simulink model "SWT_fullModel_final"  (R2023b)
settings: Solver=FixedStepAuto  StartTime=0.0  StopTime=329  RelTol=1e-3
values from neighbouring files (symbols this model uses):
  A = 19.76    [init_SWT_final.m]
  alpha = 0.19    [init_SWT_final.m]
  Cf = 1e-6    (= 1e-06)    [init_SWT_final.m]
  Cg_half = 36e-6    (= 3.6e-05)    [init_SWT_final.m]
  Cp_half = 0.8e-6    (= 8e-07)    [init_SWT_final.m]
  D_eq = 1500    [init_SWT_final.m]
  gearbox_ratio = 8.27    [init_SWT_final.m]
  J_g = 0.0491    [init_SWT_final.m]
  J_r = 142.99    [init_SWT_final.m]
  K_eq = 16887    [init_SWT_final.m]
  Lg = 12e-3    (= 0.012)    [init_SWT_final.m]
  LsLm = 3.75e-3    (= 0.00375)    [init_SWT_final.m]
  n_pp = 2    [init_SWT_final.m]
  r_rot = sqrt(A/pi)    [init_SWT_final.m]
  Rg = 2    [init_SWT_final.m]
  rho = 1.225    [init_SWT_final.m]
  Rlp1 = 100    [init_SWT_final.m]
  Rlp2 = 74    [init_SWT_final.m]
  RsRm = 2.49    [init_SWT_final.m]
  T_rated = n_eff_gen*5800/w_r_rated    [init_SWT_final.m]
  Ug = 400    [init_SWT_final.m]
  z = 12    [init_SWT_final.m]
  z_ref = 12    [init_SWT_final.m]
libraries: spsThreePhaseSeriesRLCBranchLib x9, spsRMSLib x6, spsThreePhaseVIMeasurementLib x4, spsGroundLib x3, dspstat3 x3, spsPower3phInstantaneousLib x3, spsSeriesRLCBranchLib x2, spsThreePhaseParallelRLCLoadLib x2, simulink x2, spsAsynchronousMachineSIUnitsLib x1, spsThreePhaseSourceLib x1, spspowerguiLib x1
settings Model: Creator=leons  LastModifiedBy=leons
settings DataIOCC: LoggingToFile=on

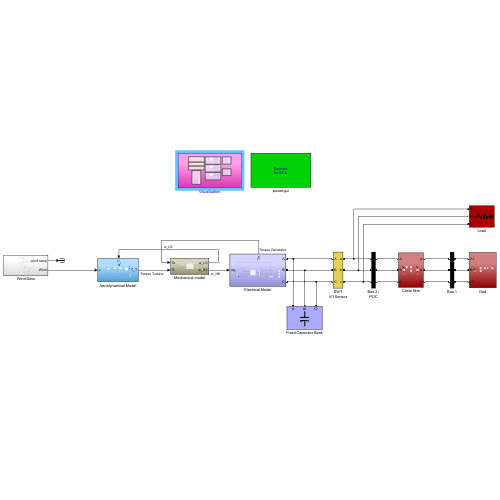
[thumbnail: Simulink's stored preview of the top-level diagram]
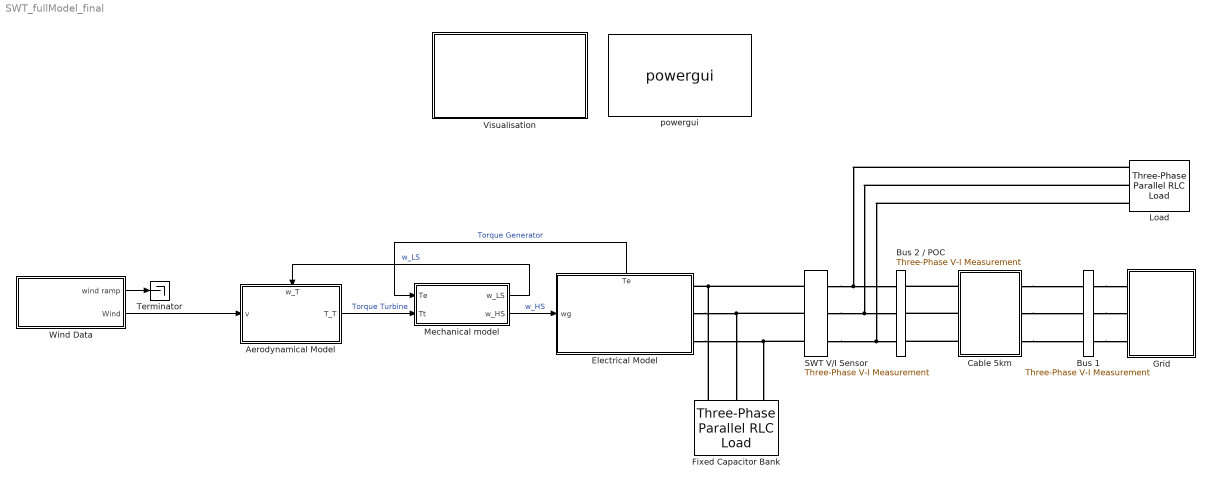
== system SWT_fullModel_final ==
  Aerodynamical Model : Subsystem
      settings: PortSchema="{\"entries\":[{\"content\":{\"sides\":[{\"content\":{\"connectorIds\":[\"In1\"]},\"type\":\"ConnectorPlacement.EquallySpacedRectSide\",\"uuid\":\"ecf32035-92b1-4f8a-b97d-d3e4d481fbcb\"},{\"content\":{\"connectorIds\":[\"Out1\"],\"side\":\"RIGHT\"},\"type\":\"ConnectorPlacement.EquallySpacedRectSide\",\"uuid\":\"1e721a83-f5e0-4c63-8c71-e92131e65c4e\"},{\"content\":{\"connectorIds\":[\"In2\"],\"side\":\"TOP\"},\"type\":\"ConnectorPlacement.EquallySpacedRectSide\",\"uuid\":\"951b011d-70ba-4a70-99b1-ab34aaa137eb\"}]},\"type\":\"ConnectorPlacement.EquallySpacedConnector\",\"uuid\":\"fe5cab3d-0189-4813-bb49-ec0d1ef7e469\"}],\"packageUris\":[\"http://schema.mathworks.com/mf0/Connector/R2020b\"],\"version\":\"1.0\"}"
  Bus 1 : spsThreePhaseVIMeasurementLib/Three-Phase V-I Measurement  VoltageMeasurement=phase-to-ground  SetLabelV=on  LabelV=Vabc_bus1  Vpu=off  VpuLL=off  CurrentMeasurement=yes  SetLabelI=on  LabelI=Iabc_bus1  Ipu=off  Pbase=100e6  Vbase=500e3  OutputType=Complex  PhasorSimulation=off  PSBequivalent=0
  Bus 2 / POC : spsThreePhaseVIMeasurementLib/Three-Phase V-I Measurement  VoltageMeasurement=phase-to-ground  SetLabelV=on  LabelV=Vabc_bus2  Vpu=off  VpuLL=off  CurrentMeasurement=yes  SetLabelI=on  LabelI=Iabc_bus2  Ipu=off  Pbase=100e6  Vbase=500e3  OutputType=Complex  PhasorSimulation=off  PSBequivalent=0
  Cable 5km : Subsystem
  Electrical Model : Subsystem
      settings: PortSchema="{\"entries\":[{\"content\":{\"sides\":[{\"content\":{\"connectorIds\":[\"In1\"]},\"type\":\"ConnectorPlacement.EquallySpacedRectSide\",\"uuid\":\"9f37345d-f4a4-45e1-920f-d9c37b4ca0b7\"},{\"content\":{\"connectorIds\":[\"RConn1\",\"RConn2\",\"RConn3\"],\"side\":\"RIGHT\"},\"type\":\"ConnectorPlacement.EquallySpacedRectSide\",\"uuid\":\"4b2a57c5-bb37-44b9-8bd5-b50d4c851d22\"},{\"content\":{\"connectorIds\":[\"Out1\"],\"side\":\"TOP\"},\"type\":\"ConnectorPlacement.EquallySpacedRectSide\",\"uuid\":\"91cf862d-bae5-40ba-b973-5330e4f84dcc\"}]},\"type\":\"ConnectorPlacement.EquallySpacedConnector\",\"uuid\":\"d5ba1b97-1505-48bd-9b20-6cd61836b2e9\"}],\"packageUris\":[\"http://schema.mathworks.com/mf0/Connector/R2020b\"],\"version\":\"1.0\"}"
  Fixed Capacitor Bank : spsThreePhaseParallelRLCLoadLib/Three-Phase Parallel RLC Load  LConnTagsString=A|B|C  Configuration=Delta  NominalVoltage=V_nominal  Vabc=[1e3 1e3 1e3]  Vabcp=[1e3 1e3 1e3]  NominalFrequency=fs  UnbalancedPower=off  ActivePower=0  InductivePower=0  CapacitivePower=Q_comp_real  Pabc=[10e3 9e3 11e3]  QLabc=[100 90 110]  QCabc=[100 90 110]  Pabcp=[10e3 9e3 11e3]  QLabcp=[100 90 110]  QCabcp=[100 90 110]  Measurements=None  LoadType=constant Z
  Grid : Subsystem
  Load : spsThreePhaseParallelRLCLoadLib/Three-Phase Parallel RLC Load  LConnTagsString=A|B|C  Configuration=Y (grounded)  NominalVoltage=400  Vabc=[1e3 1e3 1e3]  Vabcp=[1e3 1e3 1e3]  NominalFrequency=50  UnbalancedPower=off  ActivePower=Load_at_POC  InductivePower=0  CapacitivePower=0  Pabc=[10e3 9e3 11e3]  QLabc=[100 90 110]  QCabc=[100 90 110]  Pabcp=[10e3 9e3 11e3]  QLabcp=[100 90 110]  QCabcp=[100 90 110]  Measurements=None  LoadType=constant Z
  Mechanical model : Subsystem
  SWT V/I Sensor : spsThreePhaseVIMeasurementLib/Three-Phase V-I Measurement  VoltageMeasurement=phase-to-ground  SetLabelV=on  LabelV=Vabc_SWT  Vpu=off  VpuLL=off  CurrentMeasurement=yes  SetLabelI=on  LabelI=Iabc_SWT  Ipu=off  Pbase=100e6  Vbase=500e3  OutputType=Complex  PhasorSimulation=off  PSBequivalent=0
  Terminator : Terminator
  Visualisation : Subsystem
  Wind Data : Subsystem
  powergui : spspowerguiLib/powergui  Priority=1  SimulationMode=Discrete  SampleTime=50e-6  frequency=60  Iterations=50  frequencyindice=50  Pbase=100e6  ErrMax=1e-4  UnitsV=kV  UnitsW=MW  buscounter=2  FunctionMessages=off  echomessages=off  EnableUseOfTLC=off  CurrentSourceSwitches=off  DisableSnubberDevices=off  DisableRonSwitches=off  DisableVfSwitches=off  DisplayEquations=off  AutomaticDiscreteSolvers=off  SolverType=Tustin/Backward Euler (TBE)  Interpol=off  ExternalGateDelay=off  methode=off  Ts=100  x0status=blocks  SPID=on  SwTol=0  HookPort=off  NonlinearTolerance=1e-4  nMaxIteration=100  ContinueOnMaxIteration=off  RestoreLinks=warning  ResistiveCurrentMeasurement=off  Frange=[0:2:500]  Ylog=off  Xlog=on  ShowGrid=off  save=off  variable=ZData  structure=0  ZoomFFT=off  StartTime=0.0  cycles=1  DisplayStyle=1  fundamental=60  FreqAxis=off  MaxFrequency=1000  frequencyindicesteady=1  RmsSteady=1  display=off
  wires:
  Mechanical model/1(w_LS) -> Aerodynamical Model/2(w_T)  "w_LS"
  Aerodynamical Model/1(T_T) -> Mechanical model/2(Tt)  "Torque Turbine"
  Mechanical model/2(w_HS) -> Electrical Model/1(wg)  "w_HS"
  Electrical Model/1("Te ") -> Mechanical model/1(Te)  "Torque Generator"
  Wind Data/2(Wind) -> Aerodynamical Model/1(v)
  Wind Data/1(wind ramp) -> Terminator/1
  connections:
  Electrical Model/RConn3 -- Fixed Capacitor Bank/LConn3 -- SWT V/I Sensor/LConn3
  Load/LConn2 -- Bus 2 / POC/LConn2 -- SWT V/I Sensor/RConn2
  Load/LConn1 -- Bus 2 / POC/LConn1 -- SWT V/I Sensor/RConn1
  Bus 1/RConn1 -- Grid/LConn1
  Bus 1/RConn2 -- Grid/LConn2
  Bus 1/RConn3 -- Grid/LConn3
  Load/LConn3 -- SWT V/I Sensor/RConn3 -- Bus 2 / POC/LConn3
  Electrical Model/RConn2 -- Fixed Capacitor Bank/LConn2 -- SWT V/I Sensor/LConn2
  Fixed Capacitor Bank/LConn1 -- SWT V/I Sensor/LConn1 -- Electrical Model/RConn1
  Cable 5km/RConn1 -- Bus 1/LConn1
  Cable 5km/RConn2 -- Bus 1/LConn2
  Cable 5km/RConn3 -- Bus 1/LConn3
  Cable 5km/LConn1 -- Bus 2 / POC/RConn1
  Cable 5km/LConn2 -- Bus 2 / POC/RConn2
  Cable 5km/LConn3 -- Bus 2 / POC/RConn3

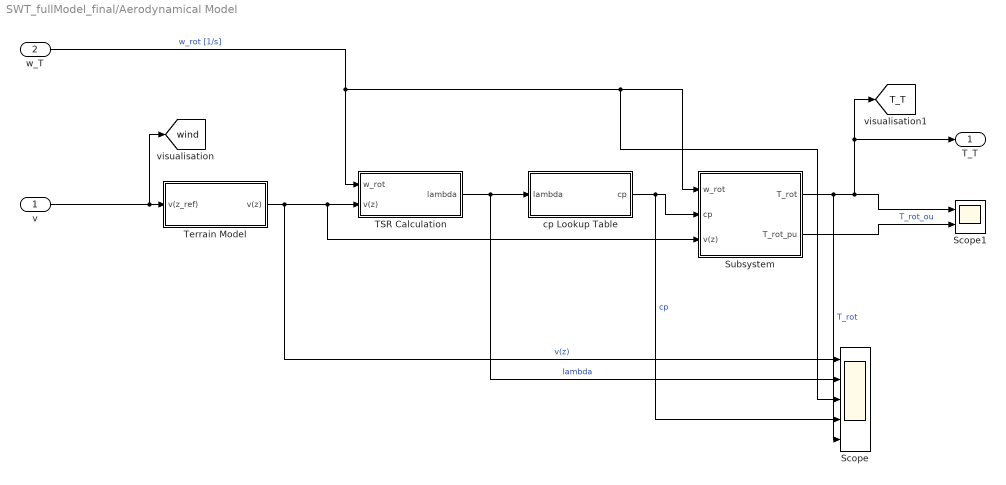
== system SWT_fullModel_final/Aerodynamical Model ==
  v : Inport
  w_T : Inport  Port=2
  Scope : Scope  NumInputPorts=5
  Scope1 : Scope  NumInputPorts=2
  Subsystem : Subsystem
  TSR Calculation : Subsystem
  Terrain Model : Subsystem
  cp Lookup Table : Subsystem
  T_T : Outport
  tag scope: T_T=global, wind=global
  wires:
  Terrain Model/1(v(z)) -> Scope/1, Subsystem/3(v(z)), TSR Calculation/2(v(z))  "v(z)"
  cp Lookup Table/1(cp) -> Scope/4, Subsystem/2(cp)  "cp"
  w_T/1 -> TSR Calculation/1(w_rot), Scope/3, Subsystem/1(w_rot)  "w_rot [1/s]"
  TSR Calculation/1(lambda) -> Scope/2, cp Lookup Table/1(lambda)  "lambda"
  Subsystem/2(T_rot_pu) -> Scope1/2  "T_rot_ou"
  v/1 -> [wind], Terrain Model/1(v(z_ref))
  Subsystem/1(T_rot) -> Scope/5, [T_T], T_T/1, Scope1/1  "T_rot"

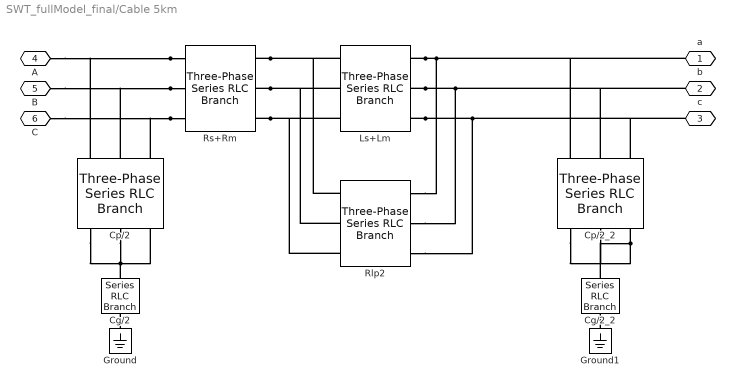
== system SWT_fullModel_final/Cable 5km ==
  Cg/2 : spsSeriesRLCBranchLib/Series RLC Branch  LConnTagsString=__new0  RConnTagsString=__new0  BranchType=C  Resistance=1  Inductance=1e-3  SetiL0=off  InitialCurrent=0  Capacitance=Cg_half  Setx0=off  InitialVoltage=0  Measurements=None
  Cg/2_2 : spsSeriesRLCBranchLib/Series RLC Branch  LConnTagsString=__new0  RConnTagsString=__new0  BranchType=C  Resistance=1  Inductance=1e-3  SetiL0=off  InitialCurrent=0  Capacitance=Cg_half  Setx0=off  InitialVoltage=0  Measurements=None
  Cp/2 : spsThreePhaseSeriesRLCBranchLib/Three-Phase Series RLC Branch  LConnTagsString=A|B|C  RConnTagsString=A|B|C  BranchType=C  Resistance=10  Inductance=12e-3  Capacitance=Cp_half  Measurements=None
  Cp/2_2 : spsThreePhaseSeriesRLCBranchLib/Three-Phase Series RLC Branch  LConnTagsString=A|B|C  RConnTagsString=A|B|C  BranchType=C  Resistance=10  Inductance=12e-3  Capacitance=Cp_half  Measurements=None
  Ground : spsGroundLib/Ground  LConnTagsString=a
  Ground1 : spsGroundLib/Ground  LConnTagsString=a
  Ls+Lm : spsThreePhaseSeriesRLCBranchLib/Three-Phase Series RLC Branch  LConnTagsString=A|B|C  RConnTagsString=A|B|C  BranchType=L  Resistance=1.28  Inductance=LsLm  Capacitance=1e-6  Measurements=None
  Rlp2 : spsThreePhaseSeriesRLCBranchLib/Three-Phase Series RLC Branch  LConnTagsString=A|B|C  RConnTagsString=A|B|C  BranchType=R  Resistance=Rlp2  Inductance=12e-3  Capacitance=1e-6  Measurements=None
  Rs+Rm : spsThreePhaseSeriesRLCBranchLib/Three-Phase Series RLC Branch  LConnTagsString=A|B|C  RConnTagsString=A|B|C  BranchType=R  Resistance=RsRm  Inductance=12e-3  Capacitance=1e-6  Measurements=None
  a : PMIOPort  Side=Right
  b : PMIOPort  Port=2  Side=Right
  c : PMIOPort  Port=3  Side=Right
  A : PMIOPort  Port=4  Side=Left
  B : PMIOPort  Port=5  Side=Left
  C : PMIOPort  Port=6  Side=Left
  connections:
  Ground1/LConn1 -- Cg/2_2/RConn1
  Cp/2_2/RConn3 -- Cg/2_2/LConn1 -- Cp/2_2/RConn2 -- Cp/2_2/RConn1
  Ground/LConn1 -- Cg/2/RConn1
  Cp/2/RConn2 -- Cg/2/LConn1 -- Cp/2/RConn3 -- Cp/2/RConn1
  Rs+Rm/LConn1 -- Cp/2/LConn1 -- A/RConn1
  Rs+Rm/LConn2 -- Cp/2/LConn2 -- B/RConn1
  Rs+Rm/LConn3 -- Cp/2/LConn3 -- C/RConn1
  Ls+Lm/RConn3 -- c/RConn1 -- Cp/2_2/LConn3 -- Rlp2/RConn3
  Ls+Lm/RConn2 -- b/RConn1 -- Cp/2_2/LConn2 -- Rlp2/RConn2
  Ls+Lm/RConn1 -- a/RConn1 -- Cp/2_2/LConn1 -- Rlp2/RConn1
  Rs+Rm/RConn3 -- Rlp2/LConn3 -- Ls+Lm/LConn3
  Rs+Rm/RConn2 -- Rlp2/LConn2 -- Ls+Lm/LConn2
  Rs+Rm/RConn1 -- Rlp2/LConn1 -- Ls+Lm/LConn1

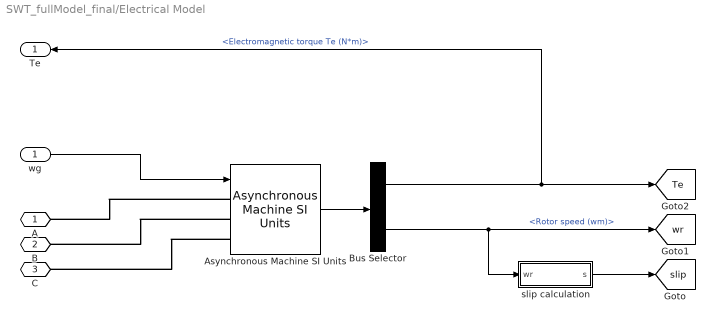
== system SWT_fullModel_final/Electrical Model ==
  wg : Inport
  Asynchronous Machine SI Units : spsAsynchronousMachineSIUnitsLib/Asynchronous Machine SI Units  RotorType=Squirrel-cage  PresetModel=No  MechanicalLoad=Speed w  ShowDetailedParameters=on  ReferenceFrame=Synchronous  Units=SI  MeasurementBus=off  NominalParameters=[5500 400 50]  VoltageRatio=1  Stator=[1.09445 0.00442]  Rotor=[1.0676 0.00442]  Cage1=[0.4155 0.002066]  Cage2=[0.4168 0.0003495]  Lm=0.14815  Mechanical=[0.0131 0.002985 2]  PolePairs=2  InitialConditions=[0 0 5.46772 5.46772 5.46772 -86.7675 -206.767 33.2325]  SimulateSaturation=off  Saturation=[14.03593122, 27.81365428, 53.79336849, 72.68890987, 97.98006896, 148.6815601, 215.7428561, 302.9841135, 428.7778367 ; 230, 322, 414, 460, 506, 552, 598, 644, 690]  LoadFlowParameters=0  TsPowergui=0  TsBlock=-1  IterativeModel=Trapezoidal non iterative  IterativeDiscreteModel=Trapezoidal non iterative  Pmec=0
  Bus Selector : BusSelector  OutputSignals=Mechanical.Electromagnetic torque Te (N*m),Mechanical.Rotor speed (wm)
  slip calculation : Subsystem
  A : PMIOPort  Side=Right
  B : PMIOPort  Port=2  Side=Right
  C : PMIOPort  Port=3  Side=Right
  "Te " : Outport
  tag scope: Te=global, slip=global, wr=global
  wires:
  Asynchronous Machine SI Units/1 -> Bus Selector/1
  wg/1 -> Asynchronous Machine SI Units/1
  Bus Selector/1 -> "Te "/1, [Te]  "<Electromagnetic torque Te (N*m)>"
  Bus Selector/2 -> slip calculation/1(wr), [wr]  "<Rotor speed (wm)>"
  slip calculation/1(s) -> [slip]
  connections:
  Asynchronous Machine SI Units/LConn2 -- B/RConn1
  Asynchronous Machine SI Units/LConn1 -- A/RConn1
  Asynchronous Machine SI Units/LConn3 -- C/RConn1

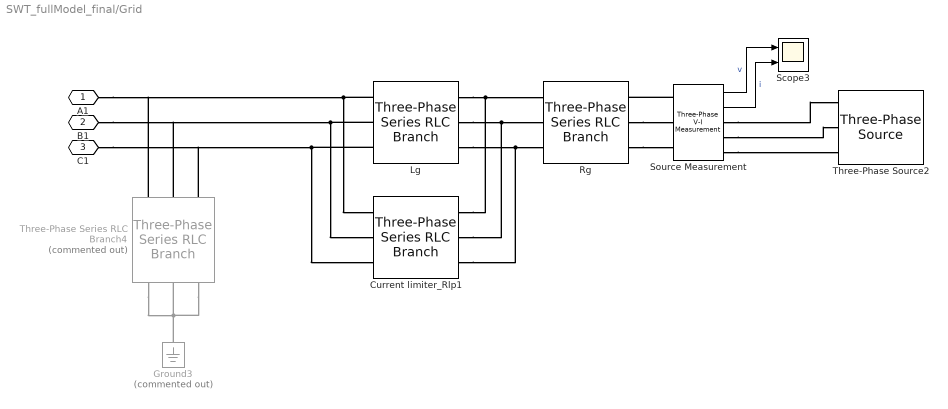
== system SWT_fullModel_final/Grid ==
  Current limiter_Rlp1 : spsThreePhaseSeriesRLCBranchLib/Three-Phase Series RLC Branch  LConnTagsString=A|B|C  RConnTagsString=A|B|C  BranchType=R  Resistance=Rlp1  Inductance=1e-3  Capacitance=1e-6  Measurements=None
  Ground3 : spsGroundLib/Ground  Commented=on  LConnTagsString=a
  Lg : spsThreePhaseSeriesRLCBranchLib/Three-Phase Series RLC Branch  LConnTagsString=A|B|C  RConnTagsString=A|B|C  BranchType=L  Resistance=200  Inductance=Lg  Capacitance=1e-6  Measurements=None
  Rg : spsThreePhaseSeriesRLCBranchLib/Three-Phase Series RLC Branch  LConnTagsString=A|B|C  RConnTagsString=A|B|C  BranchType=R  Resistance=Rg  Inductance=1e-3  Capacitance=1e-6  Measurements=None
  Scope3 : Scope  NumInputPorts=2
  Source Measurement : spsThreePhaseVIMeasurementLib/Three-Phase V-I Measurement  VoltageMeasurement=phase-to-phase  SetLabelV=off  LabelV=Vabc  Vpu=off  VpuLL=off  CurrentMeasurement=yes  SetLabelI=off  LabelI=Iabc  Ipu=off  Pbase=100e6  Vbase=500e3  OutputType=Complex  PhasorSimulation=off  PSBequivalent=0
  Three-Phase Series RLC Branch4 : spsThreePhaseSeriesRLCBranchLib/Three-Phase Series RLC Branch  Commented=on  LConnTagsString=A|B|C  RConnTagsString=A|B|C  BranchType=C  Resistance=2  Inductance=1e-3  Capacitance=Cf  Measurements=None
  Three-Phase Source2 : spsThreePhaseSourceLib/Three-Phase Source  InternalConnection=Yg  VoltagePhases=off  Voltage=Ug  PhaseAngle=0  Voltage_phases=[25e3 25e3 25e3]/sqrt(3)  PhaseAngles_phases=[0 -120 +120]  Frequency=50  NonIdealSource=off  SpecifyImpedance=off  Resistance=5.17  Inductance=12e-3  ShortCircuitLevel=100e6  BaseVoltage=400  XRratio=0.73  BusType=swing  Pref=10e3  Qref=0  Prefabc=[10e3, 10e3, 10e3]  Qrefabc=[0, 0, 0]  Qmin=-inf  Qmax=inf
  A1 : PMIOPort  Side=Left
  B1 : PMIOPort  Port=2  Side=Left
  C1 : PMIOPort  Port=3  Side=Left
  wires:
  Source Measurement/2 -> Scope3/2  "i"
  Source Measurement/1 -> Scope3/1  "v"
  connections:
  Lg/RConn2 -- Current limiter_Rlp1/RConn2 -- Rg/LConn2
  Lg/LConn1 -- Three-Phase Series RLC Branch4/LConn1 -- A1/RConn1 -- Current limiter_Rlp1/LConn1
  Lg/RConn3 -- Current limiter_Rlp1/RConn3 -- Rg/LConn3
  Lg/RConn1 -- Current limiter_Rlp1/RConn1 -- Rg/LConn1
  Lg/LConn3 -- Three-Phase Series RLC Branch4/LConn3 -- C1/RConn1 -- Current limiter_Rlp1/LConn3
  Lg/LConn2 -- Three-Phase Series RLC Branch4/LConn2 -- B1/RConn1 -- Current limiter_Rlp1/LConn2
  Source Measurement/RConn3 -- Three-Phase Source2/RConn3
  Rg/RConn2 -- Source Measurement/LConn2
  Rg/RConn3 -- Source Measurement/LConn3
  Source Measurement/RConn2 -- Three-Phase Source2/RConn2
  Source Measurement/RConn1 -- Three-Phase Source2/RConn1
  Source Measurement/LConn1 -- Rg/RConn1
  Ground3/LConn1 -- Three-Phase Series RLC Branch4/RConn3 -- Three-Phase Series RLC Branch4/RConn2 -- Three-Phase Series RLC Branch4/RConn1

== system SWT_fullModel_final/Mechanical model ==
  Te : Inport
  Tt : Inport  Port=2
  2 Mass Model : Subsystem
  Gain1 : Gain  Gain=gearbox_ratio
  Gain2 : Gain  Gain=gearbox_ratio
  Gain3 : Gain  Gain=-1
  w_LS : Outport
  w_HS : Outport  Port=2
  tag scope: w_HS=global, w_LS=global
  wires:
  Tt/1 -> 2 Mass Model/2(T_turbine)  "T_turbine"
  Te/1 -> Gain3/1  "T_generator"
  2 Mass Model/1(w_T) -> [w_LS], w_LS/1  "w_LS"
  2 Mass Model/2(w_G) -> Gain2/1
  Gain1/1 -> 2 Mass Model/1(T_generator)
  Gain3/1 -> Gain1/1
  Gain2/1 -> w_HS/1, [w_HS]  "w_HS"

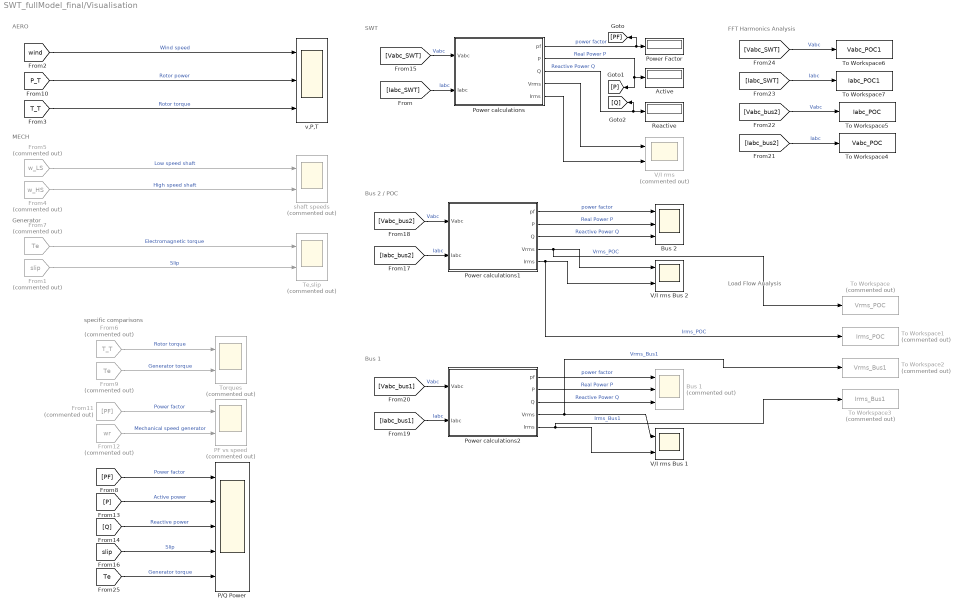
== system SWT_fullModel_final/Visualisation ==
  note: FFT Harmonics Analysis
  note: specific comparisons
  note: AERO
  note: MECH
  note: Generator
  note: SWT
  note: Bus 2 / POC
  note: Bus 1
  note: Load Flow Analysis
  Active : Display
  Bus 1 : Scope  Commented=on  NumInputPorts=3
  Bus 2 : Scope  NumInputPorts=3
  From1 : From  Commented=on  GotoTag=slip  TagVisibility=global
  From11 : From  Commented=on  GotoTag=PF
  From12 : From  Commented=on  GotoTag=wr  TagVisibility=global
  From4 : From  Commented=on  GotoTag=w_HS  TagVisibility=global
  From5 : From  Commented=on  GotoTag=w_LS  TagVisibility=global
  From6 : From  Commented=on  GotoTag=T_T  TagVisibility=global
  From7 : From  Commented=on  GotoTag=Te  TagVisibility=global
  From9 : From  Commented=on  GotoTag=Te  TagVisibility=global
  P/Q Power : Scope  NumInputPorts=5
  PF vs speed : Scope  Commented=on  NumInputPorts=2
  Power Factor : Display
  Power calculations : Subsystem
  Power calculations1 : Subsystem
  Power calculations2 : Subsystem
  Reactive : Display
  Te,slip : Scope  Commented=on  NumInputPorts=2
  To Workspace : ToWorkspace  Commented=on  VariableName=Vrms_POC  SaveFormat=Timeseries  SampleTime=1
  To Workspace1 : ToWorkspace  Commented=on  VariableName=Irms_POC  SaveFormat=Timeseries  SampleTime=1
  To Workspace2 : ToWorkspace  Commented=on  VariableName=Vrms_Bus1  SaveFormat=Timeseries  SampleTime=1
  To Workspace3 : ToWorkspace  Commented=on  VariableName=Irms_Bus1  SaveFormat=Timeseries  SampleTime=1
  To Workspace4 : ToWorkspace  VariableName=Vabc_POC  SaveFormat=Structure With Time  SampleTime=-1
  To Workspace5 : ToWorkspace  VariableName=Iabc_POC  SaveFormat=Structure With Time  SampleTime=-1
  To Workspace6 : ToWorkspace  VariableName=Vabc_POC1  SaveFormat=Structure With Time  SampleTime=-1
  To Workspace7 : ToWorkspace  VariableName=Iabc_POC1  SaveFormat=Structure With Time  SampleTime=-1
  Torques : Scope  Commented=on  NumInputPorts=2
  V/I rms : Scope  Commented=on  NumInputPorts=2
  V/I rms Bus 1 : Scope  NumInputPorts=2
  V/I rms Bus 2 : Scope  NumInputPorts=2
  shaft speeds : Scope  Commented=on  NumInputPorts=2
  v,P,T : Scope  NumInputPorts=3
  wires:
  [Vabc_SWT] -> Power calculations/1(Vabc)  "Vabc"
  [Iabc_SWT] -> Power calculations/2(Iabc)  "Iabc"
  [wind] -> v,P,T/1  "Wind speed"
  [T_T] -> v,P,T/3  "Rotor torque"
  From5/1 -> shaft speeds/1  "Low speed shaft"
  From4/1 -> shaft speeds/2  "High speed shaft"
  From7/1 -> Te,slip/1  "Electromagnetic torque"
  From1/1 -> Te,slip/2  "Slip"
  From6/1 -> Torques/1  "Rotor torque"
  From9/1 -> Torques/2  "Generator torque"
  [P_T] -> v,P,T/2  "Rotor power"
  From11/1 -> PF vs speed/1  "Power factor"
  From12/1 -> PF vs speed/2  "Mechanical speed generator"
  [PF] -> P/Q Power/1  "Power factor"
  [Q] -> P/Q Power/3  "Reactive power"
  [P] -> P/Q Power/2  "Active power"
  [slip] -> P/Q Power/4  "Slip"
  Power calculations/1(pf) -> [PF], Power Factor/1  "power factor"
  Power calculations/4(Vrms) -> V/I rms/1
  Power calculations/5(Irms) -> V/I rms/2
  Power calculations/2(P) -> Active/1, [P]  "Real Power P"
  Power calculations/3(Q) -> [Q], Reactive/1  "Reactive Power Q"
  Power calculations1/2(P) -> Bus 2/2  "Real Power P"
  Power calculations1/4(Vrms) -> To Workspace/1, V/I rms Bus 2/1  "Vrms_POC"
  Power calculations1/5(Irms) -> To Workspace1/1, V/I rms Bus 2/2  "Irms_POC"
  [Iabc_bus2] -> Power calculations1/2(Iabc)  "Iabc"
  Power calculations1/1(pf) -> Bus 2/1  "power factor"
  [Vabc_bus2] -> Power calculations1/1(Vabc)  "Vabc"
  Power calculations1/3(Q) -> Bus 2/3  "Reactive Power Q"
  [Vabc_bus1] -> Power calculations2/1(Vabc)  "Vabc"
  Power calculations2/3(Q) -> Bus 1/3  "Reactive Power Q"
  Power calculations2/1(pf) -> Bus 1/1  "power factor"
  Power calculations2/4(Vrms) -> To Workspace2/1, V/I rms Bus 1/1  "Vrms_Bus1"
  Power calculations2/5(Irms) -> To Workspace3/1, V/I rms Bus 1/2  "Irms_Bus1"
  [Iabc_bus1] -> Power calculations2/2(Iabc)  "Iabc"
  Power calculations2/2(P) -> Bus 1/2  "Real Power P"
  [Vabc_bus2] -> To Workspace5/1  "Vabc"
  [Iabc_bus2] -> To Workspace4/1  "Iabc"
  [Vabc_SWT] -> To Workspace6/1  "Vabc"
  [Iabc_SWT] -> To Workspace7/1  "Iabc"
  [Te] -> P/Q Power/5  "Generator torque"

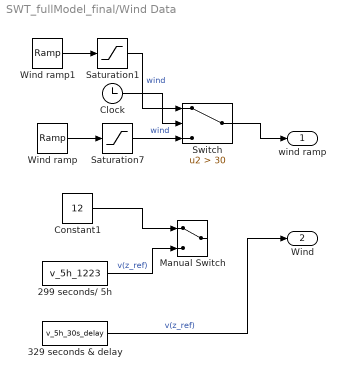
== system SWT_fullModel_final/Wind Data ==
  299 seconds/ 5h : FromWorkspace  VariableName=v_5h_1223
  329 seconds & delay : FromWorkspace  VariableName=v_5h_30s_delay
  Clock : Clock
  Constant1 : Constant  Value=12
  Manual Switch : ManualSwitch
  Saturation1 : Saturate  UpperLimit=22  LowerLimit=0
  Saturation7 : Saturate  UpperLimit=3.6  LowerLimit=0
  Switch : Switch  Criteria=u2 > Threshold  Threshold=30  SaturateOnIntegerOverflow=off  InputSameDT=off
  Wind ramp : simulink/Sources/Ramp  slope=0.25  start=0  InitialOutput=0
  Wind ramp1 : simulink/Sources/Ramp  slope=0.25  start=30  InitialOutput=3.6
  wind ramp : Outport
  Wind : Outport  Port=2
  wires:
  299 seconds/ 5h/1 -> Manual Switch/2  "v(z_ref)"
  Wind ramp/1 -> Saturation7/1
  Constant1/1 -> Manual Switch/1
  329 seconds & delay/1 -> Wind/1  "v(z_ref)"
  Clock/1 -> Switch/2
  Saturation7/1 -> Switch/3  "wind"
  Wind ramp1/1 -> Saturation1/1
  Saturation1/1 -> Switch/1  "wind"
  Switch/1 -> wind ramp/1

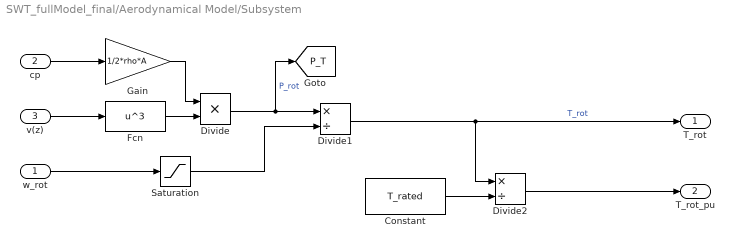
== system SWT_fullModel_final/Aerodynamical Model/Subsystem ==
  w_rot : Inport
  cp : Inport  Port=2
  v(z) : Inport  Port=3
  Constant : Constant  Value=T_rated
  Divide : Product  Inputs=**
  Divide1 : Product  Inputs=*/
  Divide2 : Product  Inputs=*/
  Fcn : Fcn  Expr=u^3
  Gain : Gain  Gain=1/2*rho*A
  Saturation : Saturate  UpperLimit=inf  LowerLimit=0.000000001
  T_rot : Outport
  T_rot_pu : Outport  Port=2
  tag scope: P_T=global
  wires:
  cp/1 -> Gain/1
  v(z)/1 -> Fcn/1
  w_rot/1 -> Saturation/1
  Divide1/1 -> Divide2/1, T_rot/1  "T_rot"
  Gain/1 -> Divide/1
  Fcn/1 -> Divide/2
  Divide/1 -> [P_T], Divide1/1  "P_rot"
  Constant/1 -> Divide2/2
  Divide2/1 -> T_rot_pu/1
  Saturation/1 -> Divide1/2

== system SWT_fullModel_final/Aerodynamical Model/TSR Calculation ==
  w_rot : Inport
  v(z) : Inport  Port=2
  Divide : Product  Inputs=*/
  Gain : Gain  Gain=r_rot
  do not divide by 0 : Saturate  UpperLimit=inf  LowerLimit=0.000000000000001
  lambda : Outport
  wires:
  w_rot/1 -> Gain/1
  Gain/1 -> Divide/1
  v(z)/1 -> do not divide by 0/1
  do not divide by 0/1 -> Divide/2
  Divide/1 -> lambda/1

== system SWT_fullModel_final/Aerodynamical Model/Terrain Model ==
  v(z_ref) : Inport
  Manual Switch : ManualSwitch
  v at measurement mast to v at nacel : Gain  Gain=(z/z_ref)^(alpha)
  z_ref = z : Gain
  v(z) : Outport
  wires:
  v at measurement mast to v at nacel/1 -> Manual Switch/1
  v(z_ref)/1 -> z_ref = z/1, v at measurement mast to v at nacel/1
  z_ref = z/1 -> Manual Switch/2
  Manual Switch/1 -> v(z)/1

== system SWT_fullModel_final/Aerodynamical Model/cp Lookup Table ==
  lambda : Inport
  Constant : Constant  Value=0
  Constant1 : Constant  Value=0
  Lambda to cp look up (w_LS varible) : Lookup_n-D  NumberOfTableDimensions=1  BreakpointsForDimension1=[2.481669207;2.539127611;2.602831328;2.677599632;2.754780313;2.834794192;2.917803625;3.005118834;3.095670955;3.187710424;3.291549784;3.405883856;3.523307507;3.648523774;3.785757295;3.931161093;4.089425538;4.25964844;4.445633778;4.648326096;4.871321625;5.118615057;5.391518918;5.693911577;6.03131319;6.412159186;6.85266606;7.369235378;7.972988668;8.687258887;9.545874399;10.59703118;11.91346096;13.61082505;15.87875732]  Table=[0.06;0.07;0.07;0.07;0.08;0.09;0.1;0.11;0.12;0.13;0.13;0.14;0.16;0.17;0.18;0.2;0.21;0.23;0.24;0.26;0.27;0.29;0.31;0.32;0.32;0.29;0.24;0.24;0.24;0.23;0.21;0.18;0.11;0.03;-0.04]  InternalRulePriority=Speed  RndMeth=Simplest
  Saturation : Saturate  UpperLimit=inf  LowerLimit=0
  cp curve : Scope
  cut in 3.5 m/s : Switch  Threshold=13.8  SaturateOnIntegerOverflow=off  InputSameDT=off
  cut out 18 m/s : Switch  Threshold=2.68467964  SaturateOnIntegerOverflow=off  InputSameDT=off
  cp : Outport
  wires:
  cut out 18 m/s/1 -> cp/1, cp curve/1
  Constant1/1 -> cut out 18 m/s/3
  lambda/1 -> cut out 18 m/s/2, cut in 3.5 m/s/3, cut in 3.5 m/s/2  "lambda"
  cut in 3.5 m/s/1 -> Lambda to cp look up (w_LS varible)/1
  Lambda to cp look up (w_LS varible)/1 -> Saturation/1
  Constant/1 -> cut in 3.5 m/s/1
  Saturation/1 -> cut out 18 m/s/1

== system SWT_fullModel_final/Electrical Model/slip calculation ==
  wr : Inport
  Add : Sum  Inputs=+-
  Display : Display
  Display1 : Display
  Divide : Product  Inputs=*/  RndMeth=Zero  SaturateOnIntegerOverflow=on
  Gain1 : Gain  Gain=2*pi
  Gain2 : Gain  Gain=1/n_pp
  fs : Constant  Value=50
  s : Outport
  wires:
  fs/1 -> Gain1/1
  Gain2/1 -> Display/1, Add/1, Divide/2  "ws"
  Add/1 -> Divide/1
  Divide/1 -> s/1
  wr/1 -> Display1/1, Add/2  "wr"
  Gain1/1 -> Gain2/1

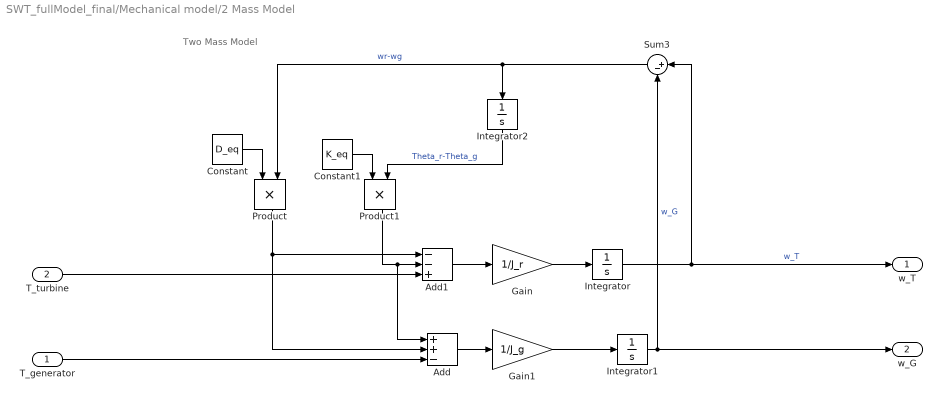
== system SWT_fullModel_final/Mechanical model/2 Mass Model ==
  note: Two Mass Model
  T_generator : Inport
  T_turbine : Inport  Port=2
  Add : Sum  Inputs=++-
  Add1 : Sum  Inputs=--+
  Constant : Constant  Value=D_eq
  Constant1 : Constant  Value=K_eq
  Gain : Gain  Gain=1/J_r
  Gain1 : Gain  Gain=1/J_g
  Integrator : Integrator
  Integrator1 : Integrator  LimitOutput=on  UpperSaturationLimit=20  LowerSaturationLimit=-20
  Integrator2 : Integrator
  Product : Product
  Product1 : Product
  Sum3 : Sum  Inputs=|+-
  w_T : Outport
  w_G : Outport  Port=2
  wires:
  Sum3/1 -> Product/2, Integrator2/1  "wr-wg"
  Product/1 -> Add/2, Add1/1
  Product1/1 -> Add/1, Add1/2
  Gain/1 -> Integrator/1
  Constant/1 -> Product/1
  Integrator1/1 -> w_G/1, Sum3/2  "w_G"
  Integrator/1 -> w_T/1, Sum3/1  "w_T"
  Integrator2/1 -> Product1/2  "Theta_r-Theta_g"
  Constant1/1 -> Product1/1
  Add/1 -> Gain1/1
  Add1/1 -> Gain/1
  T_turbine/1 -> Add1/3
  T_generator/1 -> Add/3
  Gain1/1 -> Integrator1/1

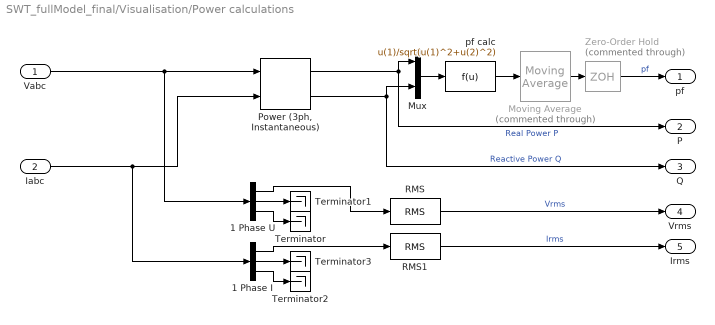
== system SWT_fullModel_final/Visualisation/Power calculations ==
  Vabc : Inport
  Iabc : Inport  Port=2
  1 Phase I : Demux  Outputs=3
  1 Phase U : Demux  Outputs=3
  Moving Average : dspstat3/Moving Average  Commented=through  Method=Sliding window  ForgettingFactorPort=off  SpecifyWindowLength=on  WindowLength=10  OverlapLength=9  AllowArbitraryInputLength=off  ForgettingFactor=0.9  SimulateUsing=Code generation
  Mux : Mux  Inputs=2
  "Power (3ph, Instantaneous)" : spsPower3phInstantaneousLib/Power (3ph, Instantaneous)
  RMS : spsRMSLib/RMS  TrueRMS=on  Freq=50  RMSInit=230  Ts=0
  RMS1 : spsRMSLib/RMS  TrueRMS=on  Freq=50  RMSInit=0  Ts=0
  Terminator{,1..3} (4 alike) : Terminator
  Zero-Order Hold : ZeroOrderHold  Commented=through  SampleTime=0.1
  pf calc : Fcn  Expr=u(1)/sqrt(u(1)^2+u(2)^2)
  pf : Outport
  P : Outport  Port=2
  Q : Outport  Port=3
  Vrms : Outport  Port=4
  Irms : Outport  Port=5
  wires:
  Mux/1 -> pf calc/1
  Moving Average/1 -> Zero-Order Hold/1
  "Power (3ph, Instantaneous)"/1 -> Mux/1, P/1  "Real Power P"
  "Power (3ph, Instantaneous)"/2 -> Mux/2, Q/1  "Reactive Power Q"
  pf calc/1 -> Moving Average/1
  Zero-Order Hold/1 -> pf/1  "pf"
  RMS1/1 -> Irms/1  "Irms"
  RMS/1 -> Vrms/1  "Vrms"
  1 Phase I/1 -> RMS1/1
  1 Phase U/3 -> Terminator/1
  Vabc/1 -> 1 Phase U/1, "Power (3ph, Instantaneous)"/1
  Iabc/1 -> 1 Phase I/1, "Power (3ph, Instantaneous)"/2
  1 Phase I/3 -> Terminator2/1
  1 Phase U/1 -> RMS/1
  1 Phase I/2 -> Terminator3/1
  1 Phase U/2 -> Terminator1/1

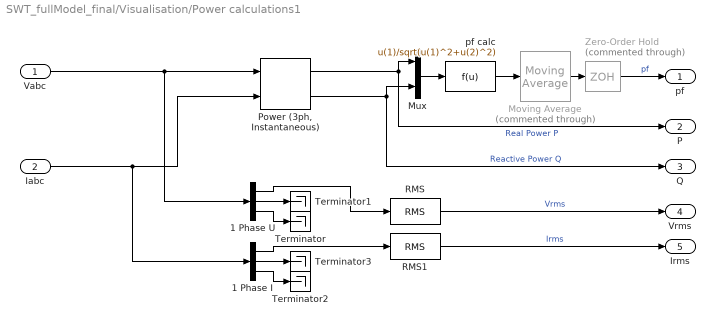
== system SWT_fullModel_final/Visualisation/Power calculations1 ==
  Vabc : Inport
  Iabc : Inport  Port=2
  1 Phase I : Demux  Outputs=3
  1 Phase U : Demux  Outputs=3
  Moving Average : dspstat3/Moving Average  Commented=through  Method=Sliding window  ForgettingFactorPort=off  SpecifyWindowLength=on  WindowLength=10  OverlapLength=9  AllowArbitraryInputLength=off  ForgettingFactor=0.9  SimulateUsing=Code generation
  Mux : Mux  Inputs=2
  "Power (3ph, Instantaneous)" : spsPower3phInstantaneousLib/Power (3ph, Instantaneous)
  RMS : spsRMSLib/RMS  TrueRMS=on  Freq=50  RMSInit=230  Ts=0
  RMS1 : spsRMSLib/RMS  TrueRMS=on  Freq=50  RMSInit=0  Ts=0
  Terminator{,1..3} (4 alike) : Terminator
  Zero-Order Hold : ZeroOrderHold  Commented=through  SampleTime=0.1
  pf calc : Fcn  Expr=u(1)/sqrt(u(1)^2+u(2)^2)
  pf : Outport
  P : Outport  Port=2
  Q : Outport  Port=3
  Vrms : Outport  Port=4
  Irms : Outport  Port=5
  wires:
  Mux/1 -> pf calc/1
  Moving Average/1 -> Zero-Order Hold/1
  "Power (3ph, Instantaneous)"/1 -> Mux/1, P/1  "Real Power P"
  "Power (3ph, Instantaneous)"/2 -> Mux/2, Q/1  "Reactive Power Q"
  pf calc/1 -> Moving Average/1
  Zero-Order Hold/1 -> pf/1  "pf"
  RMS1/1 -> Irms/1  "Irms"
  RMS/1 -> Vrms/1  "Vrms"
  1 Phase I/1 -> RMS1/1
  1 Phase U/3 -> Terminator/1
  Vabc/1 -> 1 Phase U/1, "Power (3ph, Instantaneous)"/1
  Iabc/1 -> 1 Phase I/1, "Power (3ph, Instantaneous)"/2
  1 Phase I/3 -> Terminator2/1
  1 Phase U/1 -> RMS/1
  1 Phase I/2 -> Terminator3/1
  1 Phase U/2 -> Terminator1/1

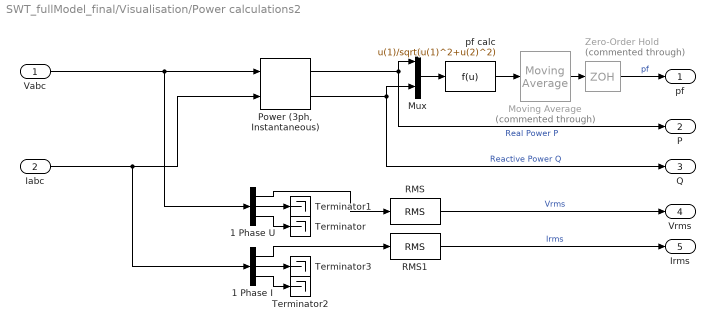
== system SWT_fullModel_final/Visualisation/Power calculations2 ==
  Vabc : Inport
  Iabc : Inport  Port=2
  1 Phase I : Demux  Outputs=3
  1 Phase U : Demux  Outputs=3
  Moving Average : dspstat3/Moving Average  Commented=through  Method=Sliding window  ForgettingFactorPort=off  SpecifyWindowLength=on  WindowLength=10  OverlapLength=9  AllowArbitraryInputLength=off  ForgettingFactor=0.9  SimulateUsing=Code generation
  Mux : Mux  Inputs=2
  "Power (3ph, Instantaneous)" : spsPower3phInstantaneousLib/Power (3ph, Instantaneous)
  RMS : spsRMSLib/RMS  TrueRMS=on  Freq=50  RMSInit=230  Ts=0
  RMS1 : spsRMSLib/RMS  TrueRMS=on  Freq=50  RMSInit=0  Ts=0
  Terminator{,1..3} (4 alike) : Terminator
  Zero-Order Hold : ZeroOrderHold  Commented=through  SampleTime=0.1
  pf calc : Fcn  Expr=u(1)/sqrt(u(1)^2+u(2)^2)
  pf : Outport
  P : Outport  Port=2
  Q : Outport  Port=3
  Vrms : Outport  Port=4
  Irms : Outport  Port=5
  wires:
  Mux/1 -> pf calc/1
  Moving Average/1 -> Zero-Order Hold/1
  "Power (3ph, Instantaneous)"/1 -> Mux/1, P/1  "Real Power P"
  "Power (3ph, Instantaneous)"/2 -> Mux/2, Q/1  "Reactive Power Q"
  pf calc/1 -> Moving Average/1
  Zero-Order Hold/1 -> pf/1  "pf"
  Iabc/1 -> 1 Phase I/1, "Power (3ph, Instantaneous)"/2
  RMS1/1 -> Irms/1  "Irms"
  RMS/1 -> Vrms/1  "Vrms"
  Vabc/1 -> 1 Phase U/1, "Power (3ph, Instantaneous)"/1
  1 Phase U/2 -> Terminator1/1
  1 Phase U/3 -> Terminator/1
  1 Phase I/3 -> Terminator2/1
  1 Phase I/2 -> Terminator3/1
  1 Phase U/1 -> RMS/1
  1 Phase I/1 -> RMS1/1
